simulink model "LOES"  (R2025b)
settings: Solver=VariableStepAuto  StartTime=0.0  StopTime=180  RelTol=1e-3
model workspace (MAT data in the model file):
  Kptheta = 0.5
values from neighbouring files (symbols this model uses):
  EngineThrustCMD = 85.0    (= 85)    [Sim6DOF_Init.m]
undefined symbols (not defined in the file or in its folder): Ktheta_LOES, Kthetdot_LOES, TF_alpha_de, TF_beta_d_ail, TF_beta_d_Rud, TF_phi_d_ail, TF_phi_d_Rud, TF_pitchrate_de, TF_psi_d_ail, TF_psi_d_Rud, TF_Theta_de, TF_u_de, TF_u_delT
libraries: simulink_extras x11, aerolibactuator x1
settings Model: Creator=Willi  LastModifiedBy=jordan

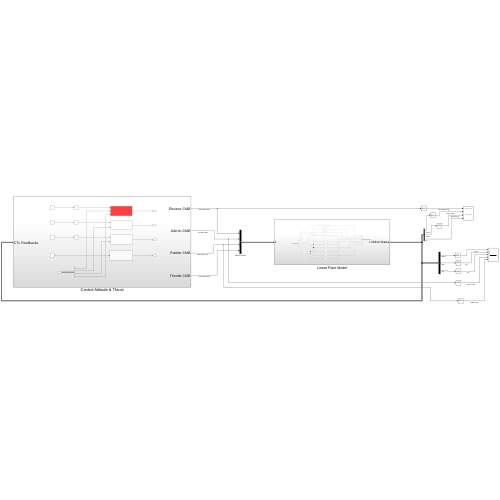
[thumbnail: Simulink's stored preview of the top-level diagram]
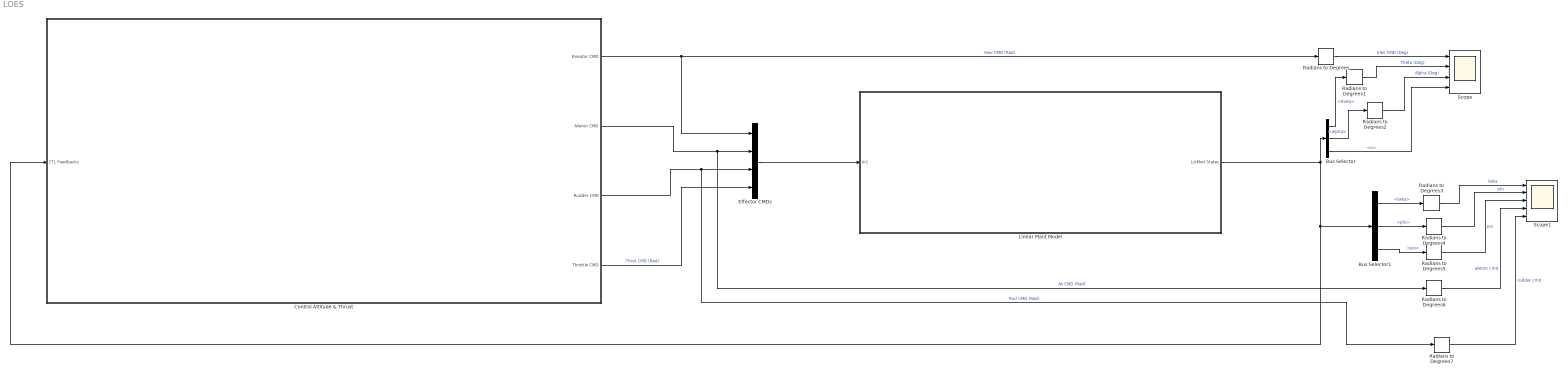
== system LOES ==
  Bus Selector : BusSelector  OutputSignals=theta,alpha,u
  Bus Selector1 : BusSelector  OutputSignals=beta,phi,psi
  Control Attitude & Thrust : Subsystem
  Effector CMDs : BusCreator  Inputs=4
  Linear Plant Model : Subsystem
  Radians to Degrees{,1..7} (8 alike) : simulink_extras/Transformations/Radians to Degrees
  Scope : Scope  NumInputPorts=4
      settings: ActiveDisplayYMinimum=-2.1486348486830908  ActiveDisplayYMaximum=11.703181649853677  DataLoggingVariableName=ScopeData12
  Scope1 : Scope  NumInputPorts=5
      settings: ActiveDisplayYMinimum=-0.020702739927473381  ActiveDisplayYMaximum=0.11083216707317123
  wires:
  Radians to Degrees4/1 -> Scope1/2  "phi"
  Radians to Degrees5/1 -> Scope1/3  "psi"
  Bus Selector/3 -> Scope/4  "<u>"
  Linear Plant Model/1(LinMod States) -> Control Attitude & Thrust/1(CTL Feedbacks), Bus Selector1/1, Bus Selector/1
  Radians to Degrees3/1 -> Scope1/1  "beta"
  Control Attitude & Thrust/2(Aileron CMD) -> Radians to Degrees6/1, Effector CMDs/2  "Ali CMD (Rad)"
  Radians to Degrees1/1 -> Scope/2  "Theta (Deg)"
  Control Attitude & Thrust/4(Throttle CMD) -> Effector CMDs/4  "Throt CMD (Rad)"
  Radians to Degrees2/1 -> Scope/3  "Alpha (Deg)"
  Radians to Degrees6/1 -> Scope1/4  "aileron cmd"
  Effector CMDs/1 -> Linear Plant Model/1(In1)
  Bus Selector1/3 -> Radians to Degrees5/1  "<psi>"
  Bus Selector/1 -> Radians to Degrees1/1  "<theta>"
  Control Attitude & Thrust/1(Elevator CMD) -> Radians to Degrees/1, Effector CMDs/1  "Elev CMD (Rad)"
  Bus Selector/2 -> Radians to Degrees2/1  "<alpha>"
  Control Attitude & Thrust/3(Rudder CMD) -> Radians to Degrees7/1, Effector CMDs/3  "Rud CMD (Rad)"
  Bus Selector1/1 -> Radians to Degrees3/1  "<beta>"
  Radians to Degrees/1 -> Scope/1  "Elev CMD (Deg)"
  Radians to Degrees7/1 -> Scope1/5  "rudder cmd"
  Bus Selector1/2 -> Radians to Degrees4/1  "<phi>"

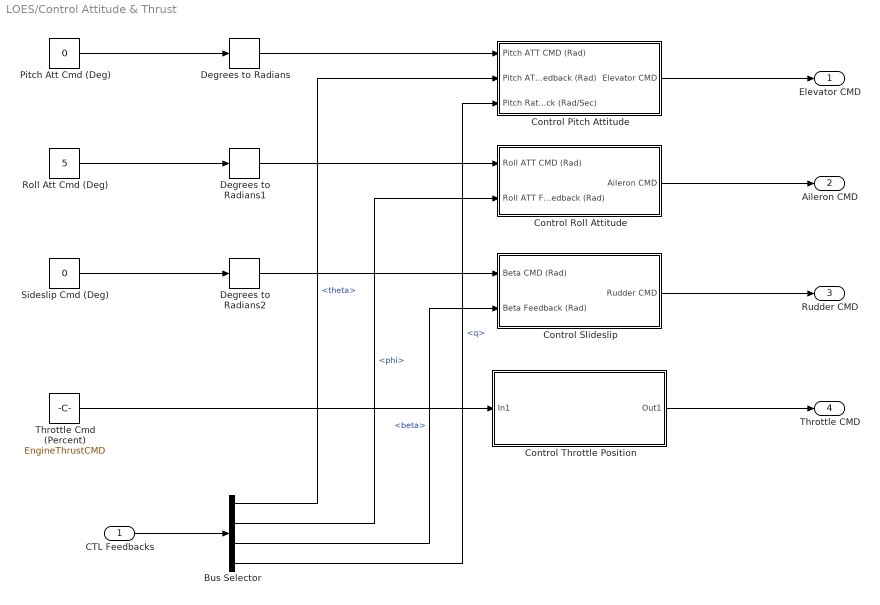
== system LOES/Control Attitude & Thrust ==
  CTL Feedbacks : Inport
  Bus Selector : BusSelector  OutputSignals=theta,phi,beta,q
  Control Pitch Attitude : Subsystem
  Control Roll Attitude : Subsystem
  Control Slideslip : Subsystem
  Control Throttle Position : Subsystem
  Degrees to Radians : simulink_extras/Transformations/Degrees to Radians
  Degrees to Radians1 : simulink_extras/Transformations/Degrees to Radians
  Degrees to Radians2 : simulink_extras/Transformations/Degrees to Radians
  Pitch Att Cmd (Deg) : Constant  Value=0
  Roll Att Cmd (Deg) : Constant  Value=5
  Sideslip Cmd (Deg) : Constant  Value=0
  Throttle Cmd (Percent) : Constant  Value=EngineThrustCMD  VectorParams1D=off
  Elevator CMD : Outport
  Aileron CMD : Outport  Port=2
  Rudder CMD : Outport  Port=3
  Throttle CMD : Outport  Port=4
  wires:
  Control Throttle Position/1(Out1) -> Throttle CMD/1
  Control Pitch Attitude/1(Elevator CMD) -> Elevator CMD/1
  Throttle Cmd (Percent)/1 -> Control Throttle Position/1(In1)
  Degrees to Radians1/1 -> Control Roll Attitude/1(Roll ATT CMD (Rad))
  Degrees to Radians2/1 -> Control Slideslip/1(Beta CMD (Rad))
  Sideslip Cmd (Deg)/1 -> Degrees to Radians2/1
  Roll Att Cmd (Deg)/1 -> Degrees to Radians1/1
  Pitch Att Cmd (Deg)/1 -> Degrees to Radians/1
  Degrees to Radians/1 -> Control Pitch Attitude/1(Pitch ATT CMD (Rad))
  CTL Feedbacks/1 -> Bus Selector/1
  Bus Selector/1 -> Control Pitch Attitude/2(Pitch ATT Feedback (Rad))  "<theta>"
  Bus Selector/2 -> Control Roll Attitude/2(Roll ATT Feedback (Rad))  "<phi>"
  Bus Selector/3 -> Control Slideslip/2(Beta Feedback (Rad))  "<beta>"
  Control Roll Attitude/1(Aileron CMD) -> Aileron CMD/1
  Control Slideslip/1(Rudder CMD) -> Rudder CMD/1
  Bus Selector/4 -> Control Pitch Attitude/3(Pitch Rate Feedback (Rad/Sec))  "<q>"

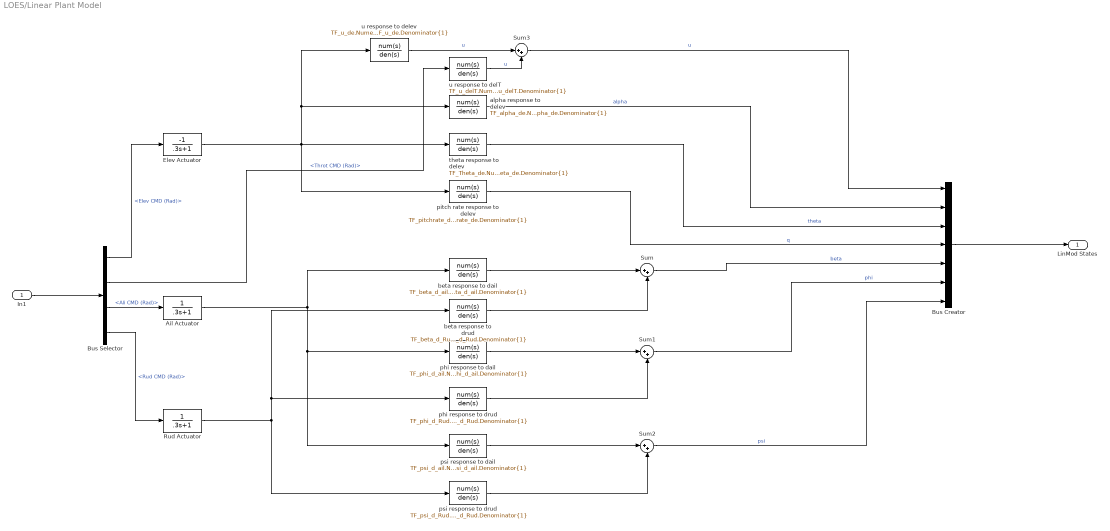
== system LOES/Linear Plant Model ==
  In1 : Inport
  " u response to delT" : TransferFcn  Numerator=TF_u_delT.Numerator{1}  Denominator=TF_u_delT.Denominator{1}
  " u response to delev" : TransferFcn  Numerator=TF_u_de.Numerator{1}  Denominator=TF_u_de.Denominator{1}
  Ail Actuator : TransferFcn  Denominator=[.3 1]
  Bus Creator : BusCreator  Inputs=7
  Bus Selector : BusSelector  OutputSignals=Elev CMD (Rad),Throt CMD (Rad),Ali CMD (Rad),Rud CMD (Rad)
  Elev Actuator : TransferFcn  Numerator=[-1]  Denominator=[.3 1]
  Rud Actuator : TransferFcn  Denominator=[.3 1]
  Sum{,1..3} (4 alike) : Sum  Inputs=|++
  alpha response to delev : TransferFcn  Numerator=TF_alpha_de.Numerator{1}  Denominator=TF_alpha_de.Denominator{1}
  beta response to dail : TransferFcn  Numerator=TF_beta_d_ail.Numerator{1}  Denominator=TF_beta_d_ail.Denominator{1}
  beta response to drud : TransferFcn  Numerator=TF_beta_d_Rud.Numerator{1}  Denominator=TF_beta_d_Rud.Denominator{1}
  phi response to dail : TransferFcn  Numerator=TF_phi_d_ail.Numerator{1}  Denominator=TF_phi_d_ail.Denominator{1}
  phi response to drud : TransferFcn  Numerator=TF_phi_d_Rud.Numerator{1}  Denominator=TF_phi_d_Rud.Denominator{1}
  pitch rate response to delev : TransferFcn  Numerator=TF_pitchrate_de.Numerator{1}  Denominator=TF_pitchrate_de.Denominator{1}
  psi response to dail : TransferFcn  Numerator=TF_psi_d_ail.Numerator{1}  Denominator=TF_psi_d_ail.Denominator{1}
  psi response to drud : TransferFcn  Numerator=TF_psi_d_Rud.Numerator{1}  Denominator=TF_psi_d_Rud.Denominator{1}
  theta response to delev : TransferFcn  Numerator=TF_Theta_de.Numerator{1}  Denominator=TF_Theta_de.Denominator{1}
  LinMod States : Outport
  wires:
  phi response to drud/1 -> Sum1/2
  beta response to drud/1 -> Sum/2
  Sum1/1 -> Bus Creator/6  "phi"
  phi response to dail/1 -> Sum1/1
  Sum2/1 -> Bus Creator/7  "psi"
  Sum/1 -> Bus Creator/5  "beta"
  beta response to dail/1 -> Sum/1
  theta response to delev/1 -> Bus Creator/3  "theta"
  Bus Creator/1 -> LinMod States/1
  psi response to dail/1 -> Sum2/1
  psi response to drud/1 -> Sum2/2
  alpha response to delev/1 -> Bus Creator/2  "alpha"
  In1/1 -> Bus Selector/1
  Sum3/1 -> Bus Creator/1  "u"
  Bus Selector/1 -> Elev Actuator/1  "<Elev CMD (Rad)>"
  Bus Selector/4 -> Rud Actuator/1  "<Rud CMD (Rad)>"
  Bus Selector/3 -> Ail Actuator/1  "<Ali CMD (Rad)>"
  Elev Actuator/1 -> pitch rate response to delev/1, " u response to delev"/1, alpha response to delev/1, theta response to delev/1
  Ail Actuator/1 -> beta response to dail/1, psi response to dail/1, phi response to dail/1
  Rud Actuator/1 -> beta response to drud/1, phi response to drud/1, psi response to drud/1
  pitch rate response to delev/1 -> Bus Creator/4  "q"
  Bus Selector/2 -> " u response to delT"/1  "<Throt CMD (Rad)>"
  " u response to delev"/1 -> Sum3/1  "u"
  " u response to delT"/1 -> Sum3/2  "u"

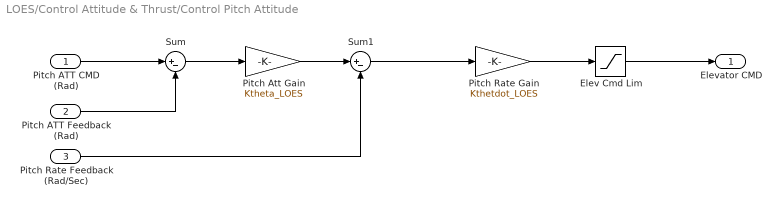
== system LOES/Control Attitude & Thrust/Control Pitch Attitude ==
  Pitch ATT CMD (Rad) : Inport
  Pitch ATT Feedback (Rad) : Inport  Port=2
  Pitch Rate Feedback (Rad/Sec) : Inport  Port=3
  Elev Cmd Lim : Saturate  UpperLimit=30  LowerLimit=-30
  Pitch Att Gain : Gain  Gain=Ktheta_LOES
  Pitch Rate Gain : Gain  Gain=Kthetdot_LOES
  Sum : Sum  Inputs=|+-
  Sum1 : Sum  Inputs=|+-
  Elevator CMD : Outport
  wires:
  Pitch ATT Feedback (Rad)/1 -> Sum/2
  Pitch ATT CMD (Rad)/1 -> Sum/1
  Sum/1 -> Pitch Att Gain/1
  Elev Cmd Lim/1 -> Elevator CMD/1
  Pitch Att Gain/1 -> Sum1/1
  Pitch Rate Feedback (Rad/Sec)/1 -> Sum1/2
  Sum1/1 -> Pitch Rate Gain/1
  Pitch Rate Gain/1 -> Elev Cmd Lim/1

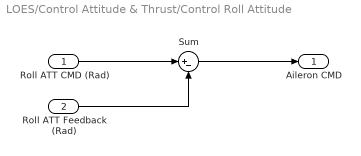
== system LOES/Control Attitude & Thrust/Control Roll Attitude ==
  Roll ATT CMD (Rad) : Inport
  Roll ATT Feedback (Rad) : Inport  Port=2
  Sum : Sum  Inputs=|+-
  Aileron CMD : Outport
  wires:
  Roll ATT CMD (Rad)/1 -> Sum/1
  Roll ATT Feedback (Rad)/1 -> Sum/2
  Sum/1 -> Aileron CMD/1

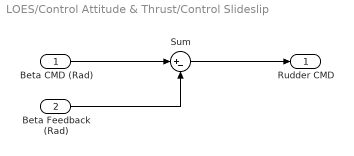
== system LOES/Control Attitude & Thrust/Control Slideslip ==
  Beta CMD (Rad) : Inport
  Beta Feedback (Rad) : Inport  Port=2
  Sum : Sum  Inputs=|+-
  Rudder CMD : Outport
  wires:
  Beta CMD (Rad)/1 -> Sum/1
  Sum/1 -> Rudder CMD/1
  Beta Feedback (Rad)/1 -> Sum/2

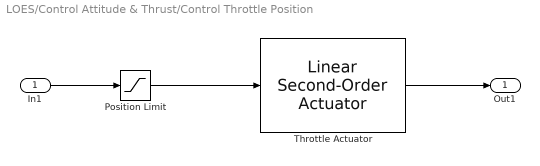
== system LOES/Control Attitude & Thrust/Control Throttle Position ==
  In1 : Inport
  Position Limit : Saturate  UpperLimit=1  LowerLimit=0
  Throttle Actuator : aerolibactuator/Linear Second-Order Actuator  wn_fin=1  z_fin=1.0  fin_act_0=EngineThrustCMD  fin_act_vel=0
  Out1 : Outport
  wires:
  In1/1 -> Position Limit/1
  Throttle Actuator/1 -> Out1/1
  Position Limit/1 -> Throttle Actuator/1
